simulink model "testing4"  (R2021a)
settings: Solver=FixedStepDiscrete  StartTime=0.0  StopTime=50  FixedStep=1  RelTol=1e-3
libraries: simulink x6
settings Model: Creator=Rahul  LastModifiedBy=Rahul

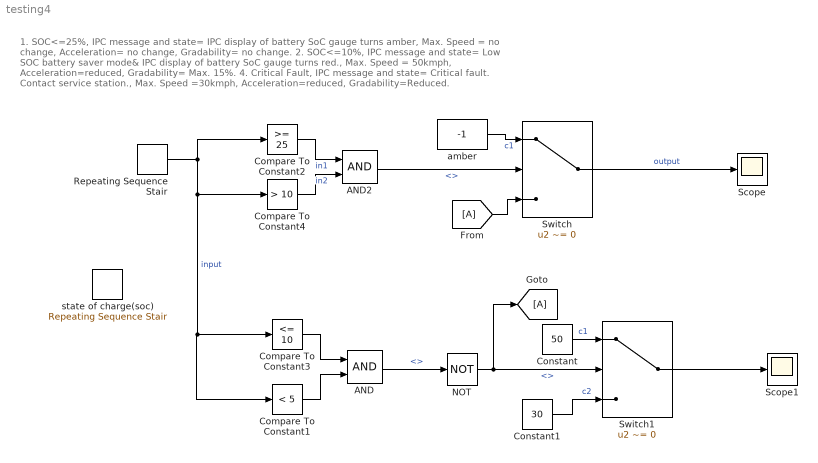
== system testing4 ==
  note: 1. SOC<=25%, IPC message and state= IPC display of battery SoC gauge turns amber, Max. Speed = no change, Acceleration= no change, Gradability= no change.
      | 2. SOC<=10%, IPC message and state= Low SOC battery saver mode& IPC display of battery SoC gauge turns red., Max. Speed = 50kmph, Acceleration=reduced, Gradability= Max. 15%.
      | 4. Critical Fault, IPC message and state= Critical fault. Contact service station., Max. Speed =30kmph, Acceleration=reduced, Gradability=Reduced.
  AND : Logic  AllPortsSameDT=off  OutDataTypeStr=boolean
  AND2 : Logic  AllPortsSameDT=off  OutDataTypeStr=boolean
  Compare To Constant1 : simulink/Logic and Bit Operations/Compare To Constant  relop=<  const=5  OutDataTypeStr=boolean
  Compare To Constant2 : simulink/Logic and Bit Operations/Compare To Constant  relop=>=  const=25  OutDataTypeStr=boolean
  Compare To Constant3 : simulink/Logic and Bit Operations/Compare To Constant  relop=<=  const=10  OutDataTypeStr=boolean
  Compare To Constant4 : simulink/Logic and Bit Operations/Compare To Constant  relop=>  const=10  OutDataTypeStr=boolean
  Constant : Constant  Value=50
  Constant1 : Constant  Value=30
  NOT : Logic  Operator=NOT  IconShape=distinctive  AllPortsSameDT=off  OutDataTypeStr=boolean
  Repeating Sequence Stair : simulink/Sources/Repeating Sequence Stair  OutValues=[9 10 4 20 30 3 40 50 12 19 25 4]  tsamp=-1  OutMin=[]  OutMax=[]  OutDataTypeStr=double  OutputDataTypeScalingMode=double  OutDataType=fixdt(0,8)  ConRadixGroup=Best Precision: Vector-wise  OutScaling=2^-12
  Scope : Scope
  Scope1 : Scope
  Switch : Switch  Criteria=u2 ~= 0
  Switch1 : Switch  Criteria=u2 ~= 0
  amber : Constant  Value=-1
  state of charge(soc) : simulink/Sources/Repeating Sequence Stair  OutValues="[9 10 4 20 30 3 40  12 19 25 50 4]"  tsamp=-1  OutMin=[]  OutMax=[]  OutDataTypeStr=double  OutputDataTypeScalingMode=double  OutDataType=fixdt(0,8)  ConRadixGroup=Best Precision: Vector-wise  OutScaling=2^-12
  wires:
  Repeating Sequence Stair/1 -> Compare To Constant2/1, Compare To Constant1/1, Compare To Constant3/1, Compare To Constant4/1  "input"
  AND2/1 -> Switch/2  "<>"
  Compare To Constant2/1 -> AND2/1  "in1"
  Compare To Constant4/1 -> AND2/2  "in2"
  Compare To Constant1/1 -> AND/2
  AND/1 -> NOT/1  "<>"
  Compare To Constant3/1 -> AND/1
  NOT/1 -> [A], Switch1/2  "<>"
  [A] -> Switch/3
  amber/1 -> Switch/1  "c1"
  Switch/1 -> Scope/1  "output"
  Constant/1 -> Switch1/1  "c1"
  Switch1/1 -> Scope1/1
  Constant1/1 -> Switch1/3  "c2"
